simulink model "SpeedCtrl"  (R2022b)
settings: Solver=FixedStepDiscrete  StartTime=0.0  StopTime=10.0  FixedStep=0.0001  RelTol=1e-3
undefined symbols (not defined in the file or in its folder): cSpeedLoopMode, cTorqueLoopMode, ParamCfg_MaxSpeed_u16, ParamCfg_SpeedKi_u16, ParamCfg_SpeedKp_u16
libraries: YS_UserDefined_Library x1
settings Model: DataDictionary=SpeedCtrl.sldd  Creator=ZYH  LastModifiedBy=ZYH
settings OptimizationCC: DefaultParameterBehavior=Inlined  EnhancedBackFolding=on  PassReuseOutputArgsAs=Individual arguments  ZeroExternalMemoryAtStartup=off  ZeroInternalMemoryAtStartup=off  OptimizeBlockOrder=speed  DifferentSizesBufferReuse=on  OptimizationCustomize=off  EfficientTunableParamExpr=on
settings DebuggingCC: ParameterTunabilityLossMsg=error
settings SFSimCC: MATLABDynamicMemAlloc=off
settings RTWCC: Description=Embedded Coder  SystemTargetFile=ert.tlc  GenCodeOnly=on  TemplateMakefile=ert_default_tmf
settings CodeAppCC: ForceParamTrailComments=on  IgnoreCustomStorageClasses=off  OperatorAnnotations=on  SimulinkDataObjDesc=on  SFDataObjDesc=on  InsertBlockDesc=on
settings ERTTargetCC: TargetLangStandard=C99 (ISO)  GenerateSampleERTMain=on  InlinedParameterPlacement=NonHierarchical  ERTCustomFileTemplate=example_file_process.tlc

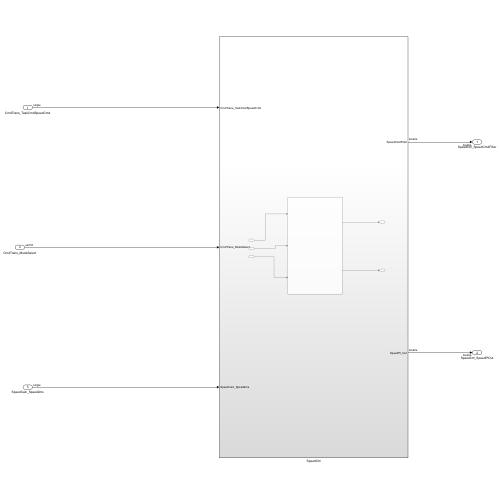
[thumbnail: Simulink's stored preview of the top-level diagram]
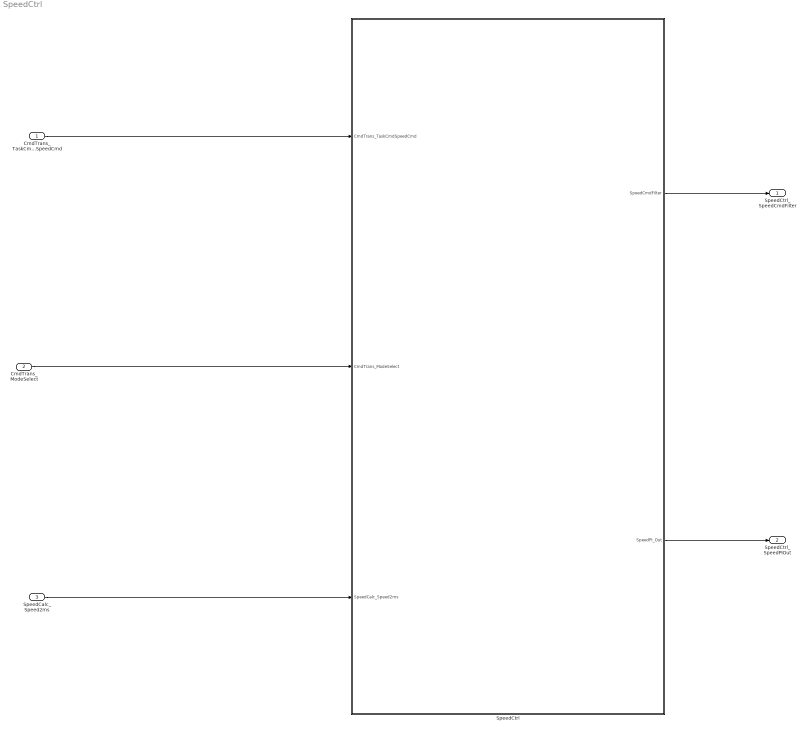
== system SpeedCtrl ==
  CmdTrans_TaskCmdSpeedCmd : Inport
  CmdTrans_ModeSelect : Inport  Port=2
  SpeedCalc_Speed2ms : Inport  Port=3
  SpeedCtrl : Subsystem
  SpeedCtrl_SpeedCmdFilter : Outport
  SpeedCtrl_SpeedPIOut : Outport  Port=2
  wires:
  CmdTrans_TaskCmdSpeedCmd/1 -> SpeedCtrl/1(CmdTrans_TaskCmdSpeedCmd)
  CmdTrans_ModeSelect/1 -> SpeedCtrl/2(CmdTrans_ModeSelect)
  SpeedCalc_Speed2ms/1 -> SpeedCtrl/3(SpeedCalc_Speed2ms)
  SpeedCtrl/1(SpeedCmdFilter) -> SpeedCtrl_SpeedCmdFilter/1
  SpeedCtrl/2(SpeedPI_Out) -> SpeedCtrl_SpeedPIOut/1

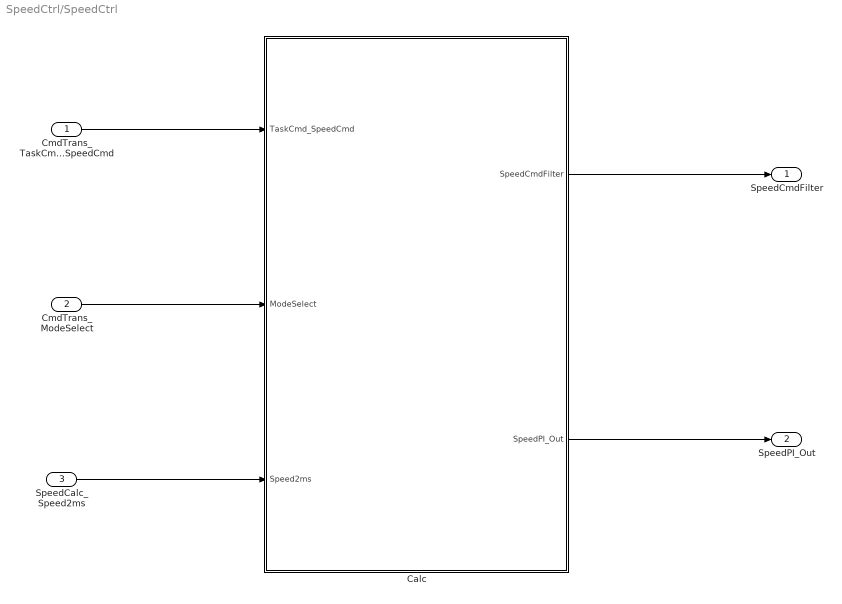
== system SpeedCtrl/SpeedCtrl ==
  CmdTrans_TaskCmdSpeedCmd : Inport
  CmdTrans_ModeSelect : Inport  Port=2
  SpeedCalc_Speed2ms : Inport  Port=3
  Calc : Subsystem
  SpeedCmdFilter : Outport
  SpeedPI_Out : Outport  Port=2
  wires:
  CmdTrans_TaskCmdSpeedCmd/1 -> Calc/1(TaskCmd_SpeedCmd)
  CmdTrans_ModeSelect/1 -> Calc/2(ModeSelect)
  SpeedCalc_Speed2ms/1 -> Calc/3(Speed2ms)
  Calc/1(SpeedCmdFilter) -> SpeedCmdFilter/1
  Calc/2(SpeedPI_Out) -> SpeedPI_Out/1

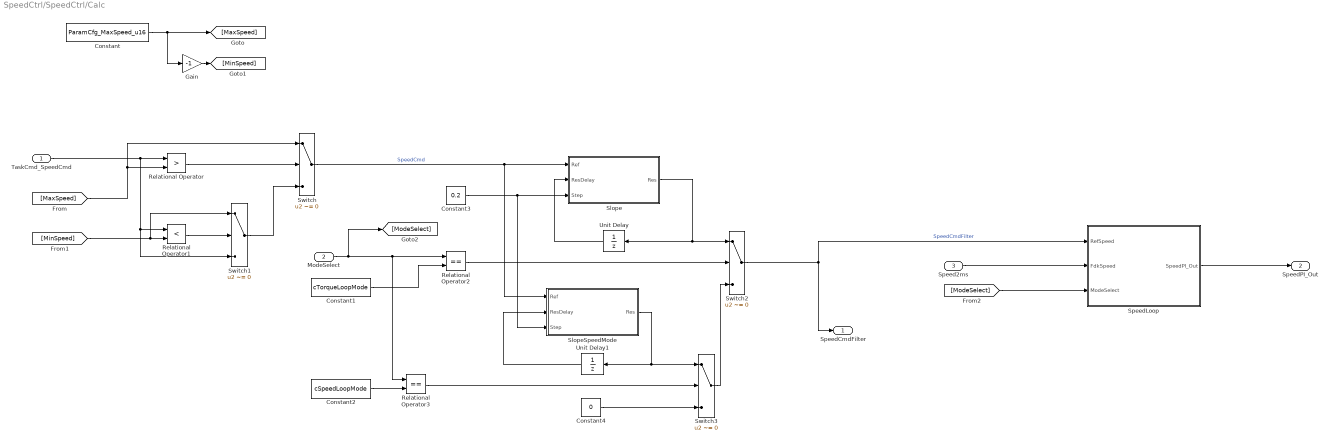
== system SpeedCtrl/SpeedCtrl/Calc ==
  TaskCmd_SpeedCmd : Inport
  ModeSelect : Inport  Port=2
  Speed2ms : Inport  Port=3
  Constant : Constant  Value=ParamCfg_MaxSpeed_u16  OutDataTypeStr=single
  Constant1 : Constant  Value=cTorqueLoopMode
  Constant2 : Constant  Value=cSpeedLoopMode
  Constant3 : Constant  Value=0.2  OutDataTypeStr=single
  Constant4 : Constant  Value=0  OutDataTypeStr=single
  Gain : Gain  Gain=-1  ParamDataTypeStr=single  OutDataTypeStr=single
  Relational Operator : RelationalOperator  Operator=>  OutDataTypeStr=boolean  RndMeth=Simplest  InputSameDT=off
  Relational Operator1 : RelationalOperator  Operator=<  OutDataTypeStr=boolean  RndMeth=Simplest  InputSameDT=off
  Relational Operator2 : RelationalOperator  Operator===  OutDataTypeStr=boolean  RndMeth=Simplest  InputSameDT=off
  Relational Operator3 : RelationalOperator  Operator===  OutDataTypeStr=boolean  RndMeth=Simplest  InputSameDT=off
  Slope : Subsystem
  SlopeSpeedMode : Subsystem
  SpeedLoop : Subsystem
  Switch{,1..3} (4 alike) : Switch  Criteria=u2 ~= 0  SaturateOnIntegerOverflow=off  InputSameDT=off
  Unit Delay : UnitDelay  SampleTime=-1  HasFrameUpgradeWarning=on
  Unit Delay1 : UnitDelay  SampleTime=-1  HasFrameUpgradeWarning=on
  SpeedCmdFilter : Outport
  SpeedPI_Out : Outport  Port=2
  wires:
  Constant/1 -> [MaxSpeed], Gain/1
  Gain/1 -> [MinSpeed]
  Relational Operator/1 -> Switch/2
  [MaxSpeed] -> Switch/1, Relational Operator/2
  TaskCmd_SpeedCmd/1 -> Switch1/3, Relational Operator1/1, Relational Operator/1
  Relational Operator1/1 -> Switch1/2
  [MinSpeed] -> Switch1/1, Relational Operator1/2
  Switch1/1 -> Switch/3
  Switch/1 -> SlopeSpeedMode/1(Ref), Slope/1(Ref)  "SpeedCmd"
  ModeSelect/1 -> [ModeSelect], Relational Operator3/1, Relational Operator2/1
  Constant1/1 -> Relational Operator2/2
  Relational Operator2/1 -> Switch2/2
  Constant2/1 -> Relational Operator3/2
  Switch2/1 -> SpeedLoop/1(RefSpeed), SpeedCmdFilter/1  "SpeedCmdFilter"
  Slope/1(Res) -> Unit Delay/1, Switch2/1
  Unit Delay/1 -> Slope/2(ResDelay)
  Constant3/1 -> SlopeSpeedMode/3(Step), Slope/3(Step)
  Relational Operator3/1 -> Switch3/2
  SlopeSpeedMode/1(Res) -> Switch3/1, Unit Delay1/1
  Unit Delay1/1 -> SlopeSpeedMode/2(ResDelay)
  Constant4/1 -> Switch3/3
  Switch3/1 -> Switch2/3
  Speed2ms/1 -> SpeedLoop/2(FdkSpeed)
  [ModeSelect] -> SpeedLoop/3(ModeSelect)
  SpeedLoop/1(SpeedPI_Out) -> SpeedPI_Out/1

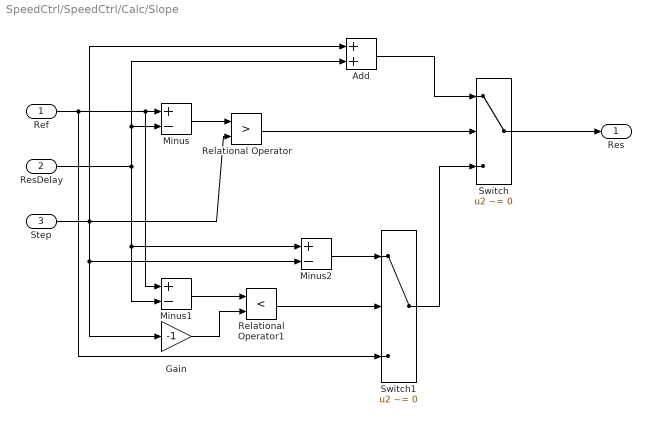
== system SpeedCtrl/SpeedCtrl/Calc/Slope ==
  Ref : Inport
  ResDelay : Inport  Port=2
  Step : Inport  Port=3
  Add : Sum
  Gain : Gain  Gain=-1  ParamDataTypeStr=single  OutDataTypeStr=single
  Minus : Sum  Inputs=+-
  Minus1 : Sum  Inputs=+-
  Minus2 : Sum  Inputs=+-
  Relational Operator : RelationalOperator  Operator=>  OutDataTypeStr=boolean  RndMeth=Simplest  InputSameDT=off
  Relational Operator1 : RelationalOperator  Operator=<  OutDataTypeStr=boolean  RndMeth=Simplest  InputSameDT=off
  Switch : Switch  Criteria=u2 ~= 0  SaturateOnIntegerOverflow=off  InputSameDT=off
  Switch1 : Switch  Criteria=u2 ~= 0  SaturateOnIntegerOverflow=off  InputSameDT=off
  Res : Outport
  wires:
  Ref/1 -> Switch1/3, Minus1/1, Minus/1
  ResDelay/1 -> Minus1/2, Minus2/1, Add/2, Minus/2
  Step/1 -> Minus2/2, Gain/1, Add/1, Relational Operator/2
  Minus/1 -> Relational Operator/1
  Relational Operator/1 -> Switch/2
  Add/1 -> Switch/1
  Minus1/1 -> Relational Operator1/1
  Gain/1 -> Relational Operator1/2
  Relational Operator1/1 -> Switch1/2
  Minus2/1 -> Switch1/1
  Switch1/1 -> Switch/3
  Switch/1 -> Res/1

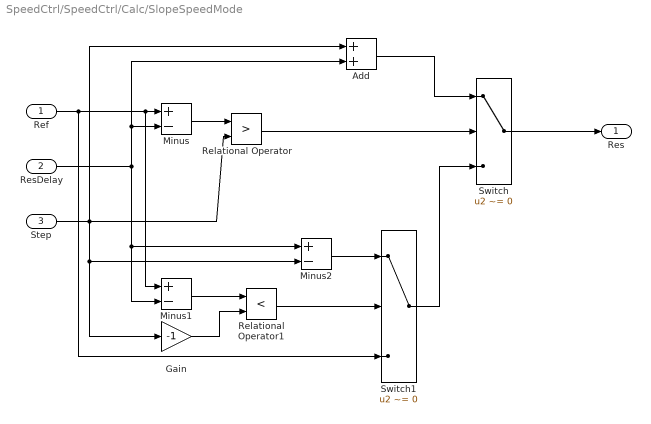
== system SpeedCtrl/SpeedCtrl/Calc/SlopeSpeedMode ==
  Ref : Inport
  ResDelay : Inport  Port=2
  Step : Inport  Port=3
  Add : Sum
  Gain : Gain  Gain=-1  ParamDataTypeStr=single  OutDataTypeStr=single
  Minus : Sum  Inputs=+-
  Minus1 : Sum  Inputs=+-
  Minus2 : Sum  Inputs=+-
  Relational Operator : RelationalOperator  Operator=>  OutDataTypeStr=boolean  RndMeth=Simplest  InputSameDT=off
  Relational Operator1 : RelationalOperator  Operator=<  OutDataTypeStr=boolean  RndMeth=Simplest  InputSameDT=off
  Switch : Switch  Criteria=u2 ~= 0  SaturateOnIntegerOverflow=off  InputSameDT=off
  Switch1 : Switch  Criteria=u2 ~= 0  SaturateOnIntegerOverflow=off  InputSameDT=off
  Res : Outport
  wires:
  Switch/1 -> Res/1
  Switch1/1 -> Switch/3
  Minus2/1 -> Switch1/1
  Relational Operator1/1 -> Switch1/2
  Gain/1 -> Relational Operator1/2
  Minus1/1 -> Relational Operator1/1
  Add/1 -> Switch/1
  Relational Operator/1 -> Switch/2
  Minus/1 -> Relational Operator/1
  Step/1 -> Relational Operator/2, Add/1, Gain/1, Minus2/2
  ResDelay/1 -> Minus/2, Add/2, Minus2/1, Minus1/2
  Ref/1 -> Minus/1, Minus1/1, Switch1/3

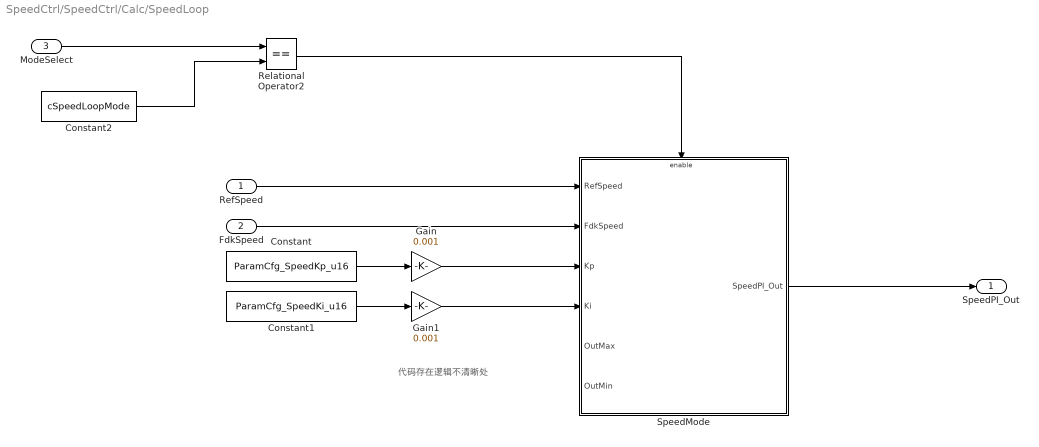
== system SpeedCtrl/SpeedCtrl/Calc/SpeedLoop ==
  note: 代码存在逻辑不清晰处
  RefSpeed : Inport
  FdkSpeed : Inport  Port=2
  ModeSelect : Inport  Port=3
  Constant : Constant  Value=ParamCfg_SpeedKp_u16
  Constant1 : Constant  Value=ParamCfg_SpeedKi_u16
  Constant2 : Constant  Value=cSpeedLoopMode
  Gain : Gain  Gain=0.001  ParamDataTypeStr=single  OutDataTypeStr=single
      settings: AttributesFormatString=%<Gain>
  Gain1 : Gain  Gain=0.001  ParamDataTypeStr=single  OutDataTypeStr=single
      settings: AttributesFormatString=%<Gain>
  Relational Operator2 : RelationalOperator  Operator===  OutDataTypeStr=boolean  RndMeth=Simplest  InputSameDT=off
  SpeedMode : Subsystem  TreatAsAtomicUnit=on
  SpeedPI_Out : Outport
  wires:
  Constant/1 -> Gain/1
  Constant1/1 -> Gain1/1
  ModeSelect/1 -> Relational Operator2/1
  Constant2/1 -> Relational Operator2/2
  Relational Operator2/1 -> SpeedMode/Enable
  Gain1/1 -> SpeedMode/4(Ki)
  Gain/1 -> SpeedMode/3(Kp)
  RefSpeed/1 -> SpeedMode/1(RefSpeed)
  FdkSpeed/1 -> SpeedMode/2(FdkSpeed)
  SpeedMode/1(SpeedPI_Out) -> SpeedPI_Out/1

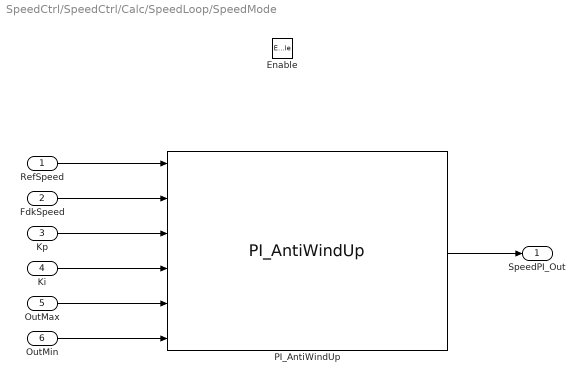
== system SpeedCtrl/SpeedCtrl/Calc/SpeedLoop/SpeedMode ==
  RefSpeed : Inport
  FdkSpeed : Inport  Port=2
  Kp : Inport  Port=3
  Ki : Inport  Port=4
  OutMax : Inport  Port=5
  OutMin : Inport  Port=6
  Enable : EnablePort
  PI_AntiWindUp : YS_UserDefined_Library/PID/PI_AntiWindUp
  SpeedPI_Out : Outport
  wires:
  RefSpeed/1 -> PI_AntiWindUp/1
  OutMin/1 -> PI_AntiWindUp/6
  OutMax/1 -> PI_AntiWindUp/5
  Ki/1 -> PI_AntiWindUp/4
  Kp/1 -> PI_AntiWindUp/3
  FdkSpeed/1 -> PI_AntiWindUp/2
  PI_AntiWindUp/1 -> SpeedPI_Out/1
